simulink model "GFLIB_ControllerPIDpAW_BAM"  (Simulink 9.3)
settings: Solver=VariableStepAuto  StartTime=0.0  StopTime=10.0  RelTol=1e-3
settings Model: Creator=nxa18952  LastModifiedBy=nxa18952
settings DataIOCC: SaveFormat=Dataset  SignalLoggingSaveFormat=Dataset  ReturnWorkspaceOutputs=on
settings OptimizationCC: LifeSpan=auto
settings DebuggingCC: UnderspecifiedInitializationDetection=Simplified  MergeDetectMultiDrivingBlocksExec=error  FcnCallInpInsideContextMsg=error  SFUnexpectedBacktrackingDiag=error  SFNoUnconditionalDefaultTransitionDiag=error  SFExecutionAtInitializationDiag=warning  ArithmeticOperatorsInVariantConditions=error
settings HardwareCC: ProdBitPerPointer=64  ProdBitPerSizeT=64  ProdBitPerPtrDiffT=64  ProdLargestAtomicFloat=Float  ProdIntDivRoundTo=Zero  ProdEndianess=LittleEndian  ProdWordSize=64  ProdHWDeviceType=Intel->x86-64 (Windows64)
settings ModelReferenceCC: PropagateSignalLabelsOutOfModel=on
settings SFSimCC: SimUseLocalCustomCode=on
settings RTWCC: RTWUseLocalCustomCode=on
settings CodeAppCC: StateflowObjectComments=off
settings GRTTargetCC: TargetLangStandard=C99 (ISO)  CombineOutputUpdateFcns=on  GRTInterface=off
settings ConfigComp: CovMetricSettings=dwe  CovHtmlReporting=off  CovSaveCumulativeToWorkspaceVar=off  CovSaveSingleToWorkspaceVar=off  CovExternalEMLEnable=on

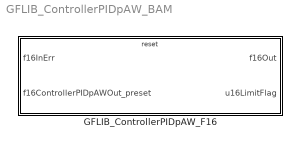
== system GFLIB_ControllerPIDpAW_BAM ==
  GFLIB_ControllerPIDpAW_F16 : Subsystem  TreatAsAtomicUnit=on  mask(GFLIB_ControllerPIDpAW_F16){showStates=Hide (faster execution), resetStatesEnable=Pre-set according to the first set of inputs after reset, f16PropGain=0, f16IntegGain=0, f16DerivGain=0, f16FiltCoef=0, s16PropGainShift=0, s16IntegGainShift=0, s16DerivGainShift=0, f16LowerLimit=0, f16UpperLimit=0}
      mask prompts: showStates "Show internal states"; resetStatesEnable "Internal state after reset"; f16PropGain "f16PropGain (Proportional gain)"; f16IntegGain "f16IntegGain (Integral gain)"; f16DerivGain "f16DerivGain (Derivative gain)"; f16FiltCoef "f16FiltCoef (Derivative term filter coefficient)"; s16PropGainShift "s16PropGainShift (Proportional gain shift)"; s16IntegGainShift "s16IntegGainShift (Integral gain shift)"; s16DerivGainShift "s16DerivGainShift (Derivative gain shift)"; f16LowerLimit "f16LowerLimit (Lower limit of the controller)"; f16UpperLimit "f16UpperLimit (Upper limit of the controller)"
      mask help: Parallel form PID controller with anti-windup in 16-bit fixed-point fractional implementation. This block supports re-initialization of the internal state during simulation. If the block is reset, the controller's output will be aligned with the input f16ControllerPIDpAWOut_preset. Refer to the AMMCLIB User's Guide for further details.
      mask init:
      | if ~evalin('base','exist(''tS8'',''var'')')
      |   if (2 ~= exist('SWLIBS_Typedefs.mat','file'))
      |       error('File SWLIBS_Typedefs.mat is not on the Matlab path. Please add the AMMCLIB "bam" folder in the Matlab Search Path.');
      |   else
      |       evalin('base', 'load(''SWLIBS_Typedefs.mat'')');
      |   end
      | end
      | if showStates == 1
      |     % hidden state variables
      |     if strcmp(get_param([gcb '/f16PropGain'], 'BlockType'), 'Inport')
      |         posblk = get_param(gcb, 'Position');
      | 
      |         pos = get_param(    [gcb, '/f16PropGain'], 'Position');
      |         orient = get_param( [gcb, '/f16PropGain'], 'Orientation');
      |         delete_block(       [gcb, '/f16PropGain']);
      |         add_block('built-in/Ground', [gcb, '/f16PropGain'], 'Position', pos, 'Orientation', orient);
      | 
      |         pos = get_param(    [gcb, '/f16IntegGain'], 'Position');
      |         orient = get_param( [gcb, '/f16IntegGain'], 'Orientation');
      |         delete_block(       [gcb, '/f16IntegGain']);
      |         add_block('built-in/Ground', [gcb, '/f16IntegGain'], 'Position', pos, 'Orientation', orient);
      | 
      |         pos = get_param(    [gcb, '/f16DerivGain'], 'Position');
      |         orient = get_param( [gcb, '/f16DerivGain'], 'Orientation');
      |         delete_block(       [gcb, '/f16DerivGain']);
      |         add_block('built-in/Ground', [gcb, '/f16DerivGain'], 'Position', pos, 'Orientation', orient);
      | 
      |         pos = get_param(    [gcb, '/f16FiltCoef'], 'Position');
      |         orient = get_param( [gcb, '/f16FiltCoef'], 'Orientation');
      |         delete_block(       [gcb, '/f16FiltCoef']);
      |         add_block('built-in/Ground', [gcb, '/f16FiltCoef'], 'Position', pos, 'Orientation', orient);
      | 
      |         pos = get_param(    [gcb, '/s16PropGainShift'], 'Position');
      |         orient = get_param( [gcb, '/s16PropGainShift'], 'Orientation');
      |         delete_block(       [gcb, '/s16PropGainShift']);
      |         add_block('built-in/Ground', [gcb, '/s16PropGainShift'], 'Position', pos, 'Orientation', orient);
      | 
      |         pos = get_param(    [gcb, '/s16IntegGainShift'], 'Position');
      |         orient = get_param( [gcb, '/s16IntegGainShift'], 'Orientation');
      |         delete_block(       [gcb, '/s16IntegGainShift']);
      |         add_block('built-in/Ground', [gcb, '/s16IntegGainShift'], 'Position', pos, 'Orientation', orient);
      | 
      |         pos = get_param(    [gcb, '/s16DerivGainShift'], 'Position');
      |         orient = get_param( [gcb, '/s16DerivGainShift'], 'Orientation');
      |         delete_block(       [gcb, '/s16DerivGainShift']);
      |         add_block('built-in/Ground', [gcb, '/s16DerivGainShift'], 'Position', pos, 'Orientation', orient);
      | 
      |         pos = get_param(    [gcb, '/f16LowerLimit'], 'Position');
      |         orient = get_param( [gcb, '/f16LowerLimit'], 'Orientation');
      |         delete_block(       [gcb, '/f16LowerLimit']);
      |         add_block('built-in/Ground', [gcb, '/f16LowerLimit'], 'Position', pos, 'Orientation', orient);
      | 
      |         pos = get_param(    [gcb, '/f16UpperLimit'], 'Position');
      |         orient = get_param( [gcb, '/f16UpperLimit'], 'Orientation');
      |         delete_block(       [gcb, '/f16UpperLimit']);
      |         add_block('built-in/Ground', [gcb, '/f16UpperLimit'], 'Position', pos, 'Orientation', orient);
      | 
      |         pos = get_param(    [gcb, '/f32IntegPartK_1'], 'Position');
      |         orient = get_param( [gcb, '/f32IntegPartK_1'], 'Orientation');
      |         delete_block(       [gcb, '/f32IntegPartK_1']);
      |         add_block('built-in/Ground', [gcb, '/f32IntegPartK_1'], 'Position', pos, 'Orientation', orient);
      | 
      |         pos = get_param(    [gcb, '/f16DerivPartK_1'], 'Position');
      |         orient = get_param( [gcb, '/f16DerivPartK_1'], 'Orientation');
      |         delete_block(       [gcb, '/f16DerivPartK_1']);
      |         add_block('built-in/Ground', [gcb, '/f16DerivPartK_1'], 'Position', pos, 'Orientation', orient);
      | 
      |         pos = get_param(    [gcb, '/f16InK_1'], 'Position');
      |         orient = get_param( [gcb, '/f16InK_1'], 'Orientation');
      |         delete_block(       [gcb, '/f16InK_1']);
      |         add_block('built-in/Ground', [gcb, '/f16InK_1'], 'Position', pos, 'Orientation', orient);
      | 
      | 
      |         pos = get_param(    [gcb '/f32IntegPartK_1_Out'], 'Position');
      |         orient = get_param( [gcb '/f32IntegPartK_1_Out'], 'Orientation');
      |         delete_block(       [gcb '/f32IntegPartK_1_Out']);
      |         add_block('built-in/Terminator', [gcb '/f32IntegPartK_1_Out'], 'Position', pos, 'Orientation', orient);
      | 
      |         pos = get_param(    [gcb '/f16DerivPartK_1_Out'], 'Position');
      |         orient = get_param( [gcb '/f16DerivPartK_1_Out'], 'Orientation');
      |         delete_block(       [gcb '/f16DerivPartK_1_Out']);
      |         add_block('built-in/Terminator', [gcb '/f16DerivPartK_1_Out'], 'Position', pos, 'Orientation', orient);
      | 
      |         pos = get_param(    [gcb '/f16InK_1_Out'], 'Position');
      |         orient = get_param( [gcb '/f16InK_1_Out'], 'Orientation');
      |         delete_block(       [gcb '/f16InK_1_Out']);
      |         add_block('built-in/Terminator', [gcb '/f16InK_1_Out'], 'Position', pos, 'Orientation', orient);
      | 
      | 
      |         set_param([gcb '/f16InErr'], 'Port', '1');
      |         set_param([gcb '/f16ControllerPIDpAWOut_preset'], 'Port', '2');
      | 
      |         set_param([gcb '/f16Out'], 'Port', '1');
      |         set_param([gcb '/u16LimitFlag'], 'Port', '2');
      | 
      |         set_param(gcb,'MaskEnables',{'on','on','on','on','on','on','on','on','on','on','on'});
      | 
      |         if (posblk(4) - posblk(2)) > 75
      |           height = 75;
      |           set_param(gcb,'Position',[posblk(1), posblk(2), posblk(3), posblk(2)+height])
      |         end
      |     end
      | else
      |     % shown state variables
      |     if strcmp(get_param([gcb '/f16PropGain'], 'BlockType'), 'Ground')
      |         posblk = get_param(gcb, 'Position');
      | 
      |         pos = get_param(    [gcb, '/f16PropGain'], 'Position');
      |         orient = get_param( [gcb, '/f16PropGain'], 'Orientation');
      |         delete_block(       [gcb, '/f16PropGain']);
      |         add_block('built-in/Inport', [gcb, '/f16PropGain'], 'Position', pos, 'Orientation', orient, 'OutDataTypeStr', 'int16');
      | 
      |         pos = get_param(    [gcb, '/f16IntegGain'], 'Position');
      |         orient = get_param( [gcb, '/f16IntegGain'], 'Orientation');
      |         delete_block(       [gcb, '/f16IntegGain']);
      |         add_block('built-in/Inport', [gcb, '/f16IntegGain'], 'Position', pos, 'Orientation', orient, 'OutDataTypeStr', 'int16');
      | 
      |         pos = get_param(    [gcb, '/f16DerivGain'], 'Position');
      |         orient = get_param( [gcb, '/f16DerivGain'], 'Orientation');
      |         delete_block(       [gcb, '/f16DerivGain']);
      |         add_block('built-in/Inport', [gcb, '/f16DerivGain'], 'Position', pos, 'Orientation', orient, 'OutDataTypeStr', 'int16');
      | 
      |         pos = get_param(    [gcb, '/f16FiltCoef'], 'Position');
      |         orient = get_param( [gcb, '/f16FiltCoef'], 'Orientation');
      |         delete_block(       [gcb, '/f16FiltCoef']);
      |         add_block('built-in/Inport', [gcb, '/f16FiltCoef'], 'Position', pos, 'Orientation', orient, 'OutDataTypeStr', 'int16');
      | 
      |         pos = get_param(    [gcb, '/s16PropGainShift'], 'Position');
      |         orient = get_param( [gcb, '/s16PropGainShift'], 'Orientation');
      |         delete_block(       [gcb, '/s16PropGainShift']);
      |         add_block('built-in/Inport', [gcb, '/s16PropGainShift'], 'Position', pos, 'Orientation', orient, 'OutDataTypeStr', 'int16');
      | 
      |         pos = get_param(    [gcb, '/s16IntegGainShift'], 'Position');
      |         orient = get_param( [gcb, '/s16IntegGainShift'], 'Orientation');
      |         delete_block(       [gcb, '/s16IntegGainShift']);
      |         add_block('built-in/Inport', [gcb, '/s16IntegGainShift'], 'Position', pos, 'Orientation', orient, 'OutDataTypeStr', 'int16');
      | 
      |         pos = get_param(    [gcb, '/s16DerivGainShift'], 'Position');
      |         orient = get_param( [gcb, '/s16DerivGainShift'], 'Orientation');
      |         delete_block(       [gcb, '/s16DerivGainShift']);
      |         add_block('built-in/Inport', [gcb, '/s16DerivGainShift'], 'Position', pos, 'Orientation', orient, 'OutDataTypeStr', 'int16');
      | 
      |         pos = get_param(    [gcb, '/f16LowerLimit'], 'Position');
      |         orient = get_param( [gcb, '/f16LowerLimit'], 'Orientation');
      |         delete_block(       [gcb, '/f16LowerLimit']);
      |         add_block('built-in/Inport', [gcb, '/f16LowerLimit'], 'Position', pos, 'Orientation', orient, 'OutDataTypeStr', 'int16');
      | 
      |         pos = get_param(    [gcb, '/f16UpperLimit'], 'Position');
      |         orient = get_param( [gcb, '/f16UpperLimit'], 'Orientation');
      |         delete_block(       [gcb, '/f16UpperLimit']);
      |         add_block('built-in/Inport', [gcb, '/f16UpperLimit'], 'Position', pos, 'Orientation', orient, 'OutDataTypeStr', 'int16');
      | 
      |         pos = get_param(    [gcb, '/f32IntegPartK_1'], 'Position');
      |         orient = get_param( [gcb, '/f32IntegPartK_1'], 'Orientation');
      |         delete_block(       [gcb, '/f32IntegPartK_1']);
      |         add_block('built-in/Inport', [gcb, '/f32IntegPartK_1'], 'Position', pos, 'Orientation', orient, 'OutDataTypeStr', 'int32');
      | 
      |         pos = get_param(    [gcb, '/f16DerivPartK_1'], 'Position');
      |         orient = get_param( [gcb, '/f16DerivPartK_1'], 'Orientation');
      |         delete_block(       [gcb, '/f16DerivPartK_1']);
      |         add_block('built-in/Inport', [gcb, '/f16DerivPartK_1'], 'Position', pos, 'Orientation', orient, 'OutDataTypeStr', 'int16');
      | 
      |         pos = get_param(    [gcb, '/f16InK_1'], 'Position');
      |         orient = get_param( [gcb, '/f16InK_1'], 'Orientation');
      |         delete_block(       [gcb, '/f16InK_1']);
      |         add_block('built-in/Inport', [gcb, '/f16InK_1'], 'Position', pos, 'Orientation', orient, 'OutDataTypeStr', 'int16');
      | 
      | 
      |         pos = get_param(    [gcb '/f32IntegPartK_1_Out'], 'Position');
      |         orient = get_param( [gcb '/f32IntegPartK_1_Out'], 'Orientation');
      |         delete_block(       [gcb '/f32IntegPartK_1_Out']);
      |         add_block('built-in/Outport', [gcb '/f32IntegPartK_1_Out'], 'Position', pos, 'Orientation', orient);
      | 
      |         pos = get_param(    [gcb '/f16DerivPartK_1_Out'], 'Position');
      |         orient = get_param( [gcb '/f16DerivPartK_1_Out'], 'Orientation');
      |         delete_block(       [gcb '/f16DerivPartK_1_Out']);
      |         add_block('built-in/Outport', [gcb '/f16DerivPartK_1_Out'], 'Position', pos, 'Orientation', orient);
      | 
      |         pos = get_param(    [gcb '/f16InK_1_Out'], 'Position');
      |         orient = get_param( [gcb '/f16InK_1_Out'], 'Orientation');
      |         delete_block(       [gcb '/f16InK_1_Out']);
      |         add_block('built-in/Outport', [gcb '/f16InK_1_Out'], 'Position', pos, 'Orientation', orient);
      | 
      | 
      |         set_param([gcb '/f16InErr'], 'Port', '1');
      |         set_param([gcb '/f16ControllerPIDpAWOut_preset'], 'Port', '2');
      |         set_param([gcb '/f16PropGain'], 'Port', '3');
      |         set_param([gcb '/f16IntegGain'], 'Port', '4');
      |         set_param([gcb '/f16DerivGain'], 'Port', '5');
      |         set_param([gcb '/f16FiltCoef'], 'Port', '6');
      |         set_param([gcb '/s16PropGainShift'], 'Port', '7');
      |         set_param([gcb '/s16IntegGainShift'], 'Port', '8');
      |         set_param([gcb '/s16DerivGainShift'], 'Port', '9');
      |         set_param([gcb '/f16LowerLimit'], 'Port', '10');
      |         set_param([gcb '/f16UpperLimit'], 'Port', '11');
      |         set_param([gcb '/f32IntegPartK_1'], 'Port', '12');
      |         set_param([gcb '/f16DerivPartK_1'], 'Port', '13');
      |         set_param([gcb '/f16InK_1'], 'Port', '14');
      | 
      |         set_param([gcb '/f16Out'], 'Port', '1');
      |         set_param([gcb '/u16LimitFlag'], 'Port', '2');
      |         set_param([gcb '/f32IntegPartK_1_Out'], 'Port', '3');
      |         set_param([gcb '/f16DerivPartK_1_Out'], 'Port', '4');
      |         set_param([gcb '/f16InK_1_Out'], 'Port', '5');
      | 
      |         set_param(gcb,'MaskEnables',{'on','on','off','off','off','off','off','off','off','off','off'});
      | 
      |         if (posblk(4) - posblk(2)) < 375
      |           height = 375;
      |           set_param(gcb,'Position',[posblk(1), posblk(2), posblk(3), posblk(2)+height])
      |         end
      |     end
      | end
      settings: RTWSystemCode=Inline
      mask TypeOptions showStates: Hide (faster execution) | Show (allows debugging; connect feedback loops manually)
      mask Callback showStates:
      | maskStr = get_param(gcb,'showStates');
      | if strcmp(maskStr,'Hide (faster execution)'),
      |     set_param(gcb,'MaskEnables',{'on','on','on','on','on','on','on','on','on','on','on'});
      | else
      |     set_param(gcb,'MaskEnables',{'on','on','off','off','off','off','off','off','off','off','off'});
      | end
      mask TypeOptions resetStatesEnable: Pre-set according to the first set of inputs after reset | Clear to zero
      mask Display:
      | color('black');
      | pos = get_param(gcb, 'Position');
      | width = pos(3) - pos(1);
      | height = pos(4) - pos(2);
      | tX=width/2;
      | tY=height - 25;
      | color('black');
      | text(tX,tY, 'GFLIB_ControllerPIDpAW_F16', 'horizontalAlignment', 'center');
      | if showStates == 2
      |   color('red');
      |   text(tX,tY - 20, ['debugging mode' char(13) char(10) '(limited performance)'], 'horizontalAlignment', 'center');
      | end

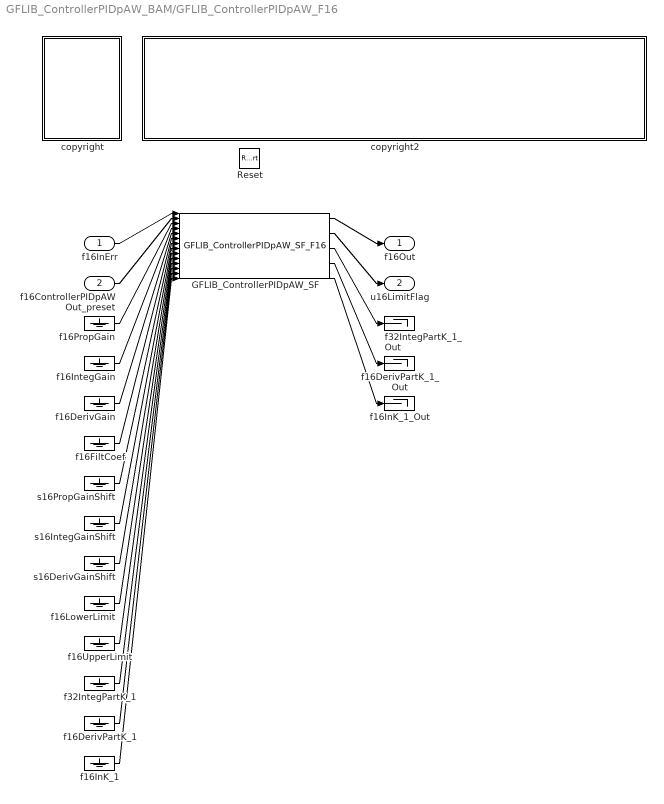
== system GFLIB_ControllerPIDpAW_BAM/GFLIB_ControllerPIDpAW_F16 ==
  f16InErr : Inport  OutDataTypeStr=int16
  f16ControllerPIDpAWOut_preset : Inport  Port=2  OutDataTypeStr=int16
  Reset : ResetPort  DisableCoverage=on
  GFLIB_ControllerPIDpAW_SF : S-Function  FunctionName=GFLIB_ControllerPIDpAW_SF_F16  Parameters=showStates,resetStatesEnable,f16PropGain,f16IntegGain,f16DerivGain,f16FiltCoef,s16PropGainShift,s16IntegGainShift,s16DerivGainShift,f16LowerLimit,f16UpperLimit  SFunctionDeploymentMode=off  EnableBusSupport=off
  copyright : Subsystem
      mask Display: text(10,90,'FILE:');text(10,75,'DESRIPTION:');text(10,60,'COPYRIGHT:');text(10,45,'VERSION:');text(10,30,'DATE:')
  copyright2 : Subsystem
      mask Display: text(10,90,'GFLIB_ControllerPIDpAW_BAM_F16.mdl');text(10,75,'Parallel form of a standard PID controller with anti-windup.');text(10,60,'NXP 2020');text(10,45,'1.0');text(10,30,'28-Mar-2020');
  f16DerivGain : Ground
  f16DerivPartK_1 : Ground
  f16DerivPartK_1_Out : Terminator
  f16FiltCoef : Ground
  f16InK_1 : Ground
  f16InK_1_Out : Terminator
  f16IntegGain : Ground
  f16LowerLimit : Ground
  f16PropGain : Ground
  f16UpperLimit : Ground
  f32IntegPartK_1 : Ground
  f32IntegPartK_1_Out : Terminator
  s16DerivGainShift : Ground
  s16IntegGainShift : Ground
  s16PropGainShift : Ground
  f16Out : Outport
  u16LimitFlag : Outport  Port=2
  wires:
  f16InErr/1 -> GFLIB_ControllerPIDpAW_SF/1
  f16ControllerPIDpAWOut_preset/1 -> GFLIB_ControllerPIDpAW_SF/2
  f16PropGain/1 -> GFLIB_ControllerPIDpAW_SF/3
  f16IntegGain/1 -> GFLIB_ControllerPIDpAW_SF/4
  f16DerivGain/1 -> GFLIB_ControllerPIDpAW_SF/5
  f16FiltCoef/1 -> GFLIB_ControllerPIDpAW_SF/6
  s16PropGainShift/1 -> GFLIB_ControllerPIDpAW_SF/7
  s16IntegGainShift/1 -> GFLIB_ControllerPIDpAW_SF/8
  s16DerivGainShift/1 -> GFLIB_ControllerPIDpAW_SF/9
  f16LowerLimit/1 -> GFLIB_ControllerPIDpAW_SF/10
  f16UpperLimit/1 -> GFLIB_ControllerPIDpAW_SF/11
  f32IntegPartK_1/1 -> GFLIB_ControllerPIDpAW_SF/12
  f16DerivPartK_1/1 -> GFLIB_ControllerPIDpAW_SF/13
  f16InK_1/1 -> GFLIB_ControllerPIDpAW_SF/14
  GFLIB_ControllerPIDpAW_SF/1 -> f16Out/1
  GFLIB_ControllerPIDpAW_SF/2 -> u16LimitFlag/1
  GFLIB_ControllerPIDpAW_SF/3 -> f32IntegPartK_1_Out/1
  GFLIB_ControllerPIDpAW_SF/4 -> f16DerivPartK_1_Out/1
  GFLIB_ControllerPIDpAW_SF/5 -> f16InK_1_Out/1

== system GFLIB_ControllerPIDpAW_BAM/GFLIB_ControllerPIDpAW_F16/copyright ==

== system GFLIB_ControllerPIDpAW_BAM/GFLIB_ControllerPIDpAW_F16/copyright2 ==
